simulink model "KD_cl_harness_cl_ouports_added"  (R2015b)
settings: Solver=ode45  StartTime=0  StopTime=inf  FixedStep=0.01  MaxStep=0.005  RelTol=1e-5  AbsTol=1e-5
undefined symbols (not defined in the file or in its folder): A2, bin_vec, c_0, c_1000, c_1000inv, c_100inv, c_1d2p4, c_1p7, c_4400inv, c_5500inv, c_80, c_compmap, c_ctok, c_fflow_max, c_fflow_min, c_filt, c_flowdiv, c_flowmin, c_flowmult, c_inf, c_km1d2k, c_n1, c_p00001, c_p01, c_p1e9, c_p4d1p4, c_pincomp, c_rair, c_roacorr, c_rpmtoradpers, c_svrthrottle1, c_svrthrottle2, c_svrthrottlearg, c_svrthrottlebeta, c_vnliftmax, c_vnliftmin, cl_offset, clff, Coefs, const, const_exhat, const_vec, Dual_array, dual_zero, egr_ecu_ff, expcon, f_mat, gs_jul, HQP_eps, HQP_INF, HQP_saturation, IV, L2, length_L, maxL, mHQP_saturation, minL, Newton, nRed, num_constraints ... (+22)
libraries: simulink x33
(part 2 of 6)

== system KD_cl_harness_cl_ouports_added/ambient_and_controls_in ==
  Bus Creator1 : BusCreator  Inputs=6
  From Workspace11 : FromWorkspace  VariableName="[0   97.4216]"  SampleTime=0  Interpolate=off  OutputAfterFinalValue=Holding final value
  From Workspace12 : FromWorkspace  VariableName="[0  296.9595]"  SampleTime=0  Interpolate=off  OutputAfterFinalValue=Holding final value
  From Workspace5 : FromWorkspace  VariableName="[0   97.4450]"  SampleTime=0  Interpolate=off  OutputAfterFinalValue=Holding final value
  From Workspace6 : FromWorkspace  VariableName="[0  300.0250]"  SampleTime=0  Interpolate=off  OutputAfterFinalValue=Holding final value
  From Workspace7 : FromWorkspace  VariableName="[0  351.4714]"  SampleTime=0  Interpolate=off  OutputAfterFinalValue=Holding final value
  From Workspace8 : FromWorkspace  VariableName="[0    3.7702]"  SampleTime=0  Interpolate=off  OutputAfterFinalValue=Holding final value
  ambient_in : Outport
  wires:
  Bus Creator1/1 -> ambient_in/1  "ambient_in"
  From Workspace11/1 -> Bus Creator1/1  "p_in_comp_data"
  From Workspace5/1 -> Bus Creator1/2  "p_ambient"
  From Workspace12/1 -> Bus Creator1/3  "T_in_comp_data"
  From Workspace6/1 -> Bus Creator1/4  "T_ambient"
  From Workspace7/1 -> Bus Creator1/5  "T_coolant"
  From Workspace8/1 -> Bus Creator1/6  "Tq_load"

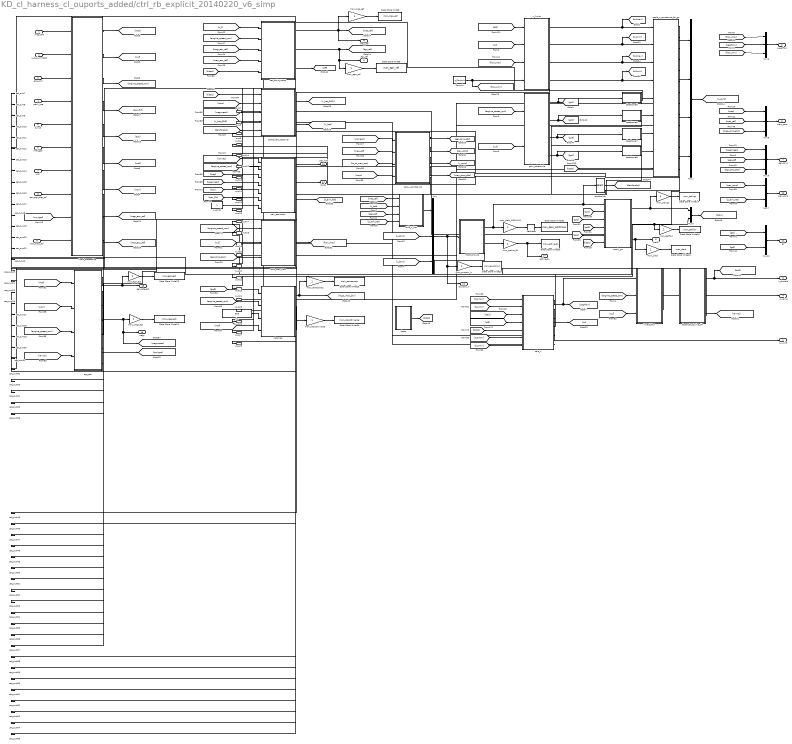
== system KD_cl_harness_cl_ouports_added/ctrl_rb_explicit_20140220_v6_simp ==
  map_kPa : Inport  OutDataTypeStr=single  PortDimensions=1  SampleTime=sample_time
  u_fuel_mm3pst : Inport  Port=2  OutDataTypeStr=single  PortDimensions=1  SampleTime=sample_time
  ene_rpm : Inport  Port=3  OutDataTypeStr=single  PortDimensions=1  SampleTime=sample_time
  pexh_kpa : Inport  Port=4  OutDataTypeStr=single  PortDimensions=1  SampleTime=sample_time
  t_in_C : Inport  Port=5  OutDataTypeStr=single  PortDimensions=1  SampleTime=sample_time
  maf_gps : Inport  Port=6  OutDataTypeStr=single  PortDimensions=1  SampleTime=sample_time
  wcyl : Inport  Port=7  OutDataTypeStr=single  PortDimensions=1  SampleTime=sample_time
  ecu_egr_rate_ref : Inport  Port=8  OutDataTypeStr=single  PortDimensions=1  SampleTime=sample_time
  ecu_map_ref : Inport  Port=9  OutDataTypeStr=single  PortDimensions=1  SampleTime=sample_time
  Data Store Write14 : DataStoreWrite  DataStoreName=mon_delvgt
  Data Store Write15 : DataStoreWrite  DataStoreName=mon_delflow
  Data Store Write16 : DataStoreWrite  DataStoreName=mon_slack
  Data Store Write23 : DataStoreWrite  DataStoreName=mon_egrr_est
  Data Store Write24 : DataStoreWrite  DataStoreName=mon_wegr_est
  Data Store Write25 : DataStoreWrite  DataStoreName=mon_remapmap
  Data Store Write29 : DataStoreWrite  DataStoreName=mon_expcon_in
  Data Store Write30 : DataStoreWrite  DataStoreName=mon_active_SL
  Data Store Write31 : DataStoreWrite  DataStoreName=mon_delU_HQPKWIK
  Data Store Write34 : DataStoreWrite  DataStoreName=mon_wtpostinverse
  Data Store Write8 : DataStoreWrite  DataStoreName=mon_map_ref
  Data Store Write9 : DataStoreWrite  DataStoreName=mon_egrr_ref
  EGR_max_flow : Subsystem
  HQPKWIK_V6 : Subsystem
  Mux{,6,8..9} (4 alike) : Mux  Inputs=3
  Mux1 : Mux
  Mux10 : Mux  Inputs=2
  Mux5 : Mux  Inputs=2
  Mux7 : Mux  Inputs=2
  Reshape : Reshape
  apply_gs : Subsystem
  calc_u : Subsystem
  calc_y_constraints : Subsystem
  constraints : Selector  InputPortWidth=3  IndexOptions=Index vector (dialog)  Indices=[1 2]  OutputSizes=1
  deadzone5 : Subsystem
  deadzone6 : Subsystem
  deadzone7 : Subsystem
  deadzone8 : Subsystem
  deconstruct_vlve_thr : Subsystem
  egr_est : Subsystem
  flowmin : Constant  Value=c_flowmin  OutDataTypeStr=single  SampleTime=sample_time
      settings: AttributesFormatString=%<Value>\n%<SampleTime>
  gain_schechule : Subsystem
  input_processing : Subsystem
  invert_flow : Subsystem  SystemSampleTime=.032
  mon_active_SL : Gain  OutDataTypeStr=int32
  mon_delU_HQPKWIK : Gain  OutDataTypeStr=single
  mon_delflow : Gain
  mon_delvgt : Gain
  mon_egrr_est : Gain
  mon_egrr_ref : Gain
  mon_expcon_in : Gain  OutDataTypeStr=single
  mon_map_ref : Gain
  mon_remapmap : Gain
  mon_slack : Gain
  mon_wegr_est : Gain
  mon_wtpostinverse : Gain
  ntremap : Subsystem  SystemSampleTime=.016
  pex_estimator : Subsystem
  scale_u_constraints_for_gs : Subsystem
  scheduled_observer : Subsystem
  set_point_maps : Subsystem
  shift_x_hat : Subsystem
  tic : Constant  Value=303  OutDataTypeStr=single  SampleTime=sample_time
      settings: AttributesFormatString=%<Value>\n%<SampleTime>
  tictoc : Subsystem
  u_limits : Subsystem
  y_cons1 : Constant  OutDataTypeStr=single  SampleTime=sample_time
      settings: AttributesFormatString=%<Value>\n%<SampleTime>
  u_vnlift : Outport  OutDataTypeStr=single
  u_egrflow : Outport  Port=2  OutDataTypeStr=single
  u_throttle : Outport  Port=3  OutDataTypeStr=single
  u_valve : Outport  Port=4  OutDataTypeStr=single
  slack : Outport  Port=5  OutDataTypeStr=single
  map_cons : Outport  Port=6  OutDataTypeStr=single
  egr_cons : Outport  Port=7  OutDataTypeStr=single
  map_ref : Outport  Port=8  OutDataTypeStr=single
  egr_ref : Outport  Port=9  OutDataTypeStr=single
  pex_cons : Outport  Port=10  OutDataTypeStr=single
  gs : Outport  Port=11  OutDataTypeStr=single
  expcon_in : Outport  Port=12  OutDataTypeStr=single
  pex_hat : Outport  Port=13  OutDataTypeStr=single
  dwdp : Outport  Port=14  OutDataTypeStr=single
  egr_rate_est : Outport  Port=15  OutDataTypeStr=single
  wegr : Outport  Port=16  OutDataTypeStr=single
  active_SL : Outport  Port=17  OutDataTypeStr=int32  PortDimensions=1
  sat_out-7 : Outport  Port=18
  sat_out-8 : Outport  Port=19
  sat_out-9 : Outport  Port=20
  sat_out-10 : Outport  Port=21
  sat_out-11 : Outport  Port=22
  sat_out-12 : Outport  Port=23
  sat_out-13 : Outport  Port=24
  sat_out-14 : Outport  Port=25
  sat_out-15 : Outport  Port=26
  sat_out-16 : Outport  Port=27
  sat_out-17 : Outport  Port=28
  sat_out-18 : Outport  Port=29
  sat_out-19 : Outport  Port=30
  sat_out-20 : Outport  Port=31
  sat_out-21 : Outport  Port=32
  sat_out-22 : Outport  Port=33
  sat_out-23 : Outport  Port=34
  sat_out-24 : Outport  Port=35
  sat_out-25 : Outport  Port=36
  sat_out-26 : Outport  Port=37
  sat_out-27 : Outport  Port=38
  sat_out-28 : Outport  Port=39
  sat_out-29 : Outport  Port=40
  sat_out-30 : Outport  Port=41
  sat_out-31 : Outport  Port=42
  sat_out-32 : Outport  Port=43
  sat_out-33 : Outport  Port=44
  sat_out-34 : Outport  Port=45
  sat_out-35 : Outport  Port=46
  sat_out-36 : Outport  Port=47
  sat_out-45 : Outport  Port=48
  sat_out-46 : Outport  Port=49
  sat_out-47 : Outport  Port=50
  sat_out-48 : Outport  Port=51
  sat_out-49 : Outport  Port=52
  sat_out-50 : Outport  Port=53
  sat_out-51 : Outport  Port=54
  sat_out-52 : Outport  Port=55
  sat_out-53 : Outport  Port=56
  sat_out-54 : Outport  Port=57
  sat_out-55 : Outport  Port=58
  sat_out-56 : Outport  Port=59
  sat_out-57 : Outport  Port=60
  sat_out-58 : Outport  Port=61
  sat_out-59 : Outport  Port=62
  sat_out-60 : Outport  Port=63
  sat_out-61 : Outport  Port=64
  sat_out-62 : Outport  Port=65
  sat_out-63 : Outport  Port=66
  sat_out-64 : Outport  Port=67
  sat_out-65 : Outport  Port=68
  out-7 : Outport  Port=69
  out-8 : Outport  Port=70
  out-9 : Outport  Port=71
  out-10 : Outport  Port=72
  out-11 : Outport  Port=73
  out-12 : Outport  Port=74
  out-13 : Outport  Port=75
  out-14 : Outport  Port=76
  out-15 : Outport  Port=77
  out-16 : Outport  Port=78
  out-17 : Outport  Port=79
  out-18 : Outport  Port=80
  out-19 : Outport  Port=81
  out-20 : Outport  Port=82
  out-21 : Outport  Port=83
  out-22 : Outport  Port=84
  out-23 : Outport  Port=85
  out-24 : Outport  Port=86
  out-25 : Outport  Port=87
  out-26 : Outport  Port=88
  out-27 : Outport  Port=89
  out-28 : Outport  Port=90
  wires:
  [tu2min] -> calc_u/7(tu2min)
  [tu2max] -> calc_u/6(tu2max)
  [tu1min] -> calc_u/2(tu1min)
  [tu1max] -> calc_u/1(tu1max)
  [wt_to_map_con] -> calc_y_constraints/3(wt_to_map_con)
  [map] -> calc_y_constraints/4(map)
  ntremap/2(wtinv) -> mon_wtpostinverse/1
  mon_wtpostinverse/1 -> Data Store Write34/1
  [map_ecu_ref] -> set_point_maps/4(map_ecu_ref)
  [wegr_ecu_ref] -> set_point_maps/3(wegr_ecu_ref)
  [wcylgps] -> input_processing/9(wcylgps)
  egr_est/3(wcylgps) -> [wcylgps]
  ecu_map_ref/1 -> input_processing/10(ecu_map_ref)
  [w_f] -> gain_schechule/2(qv)
  [engine_speed_rpm] -> gain_schechule/1(ene)
  mon_remapmap/1 -> Data Store Write25/1
  ntremap/1(mapconsremaped) -> mon_remapmap/1, [wt_to_map_con]
  [tictoc] -> calc_u/5(tictoc)
  deadzone8/1(Out1) -> scale_u_constraints_for_gs/8(gs4)
  deadzone7/1(Out1) -> scale_u_constraints_for_gs/7(gs3)
  deadzone6/1(Out1) -> scale_u_constraints_for_gs/6(gs2)
  deadzone5/1(Out1) -> scale_u_constraints_for_gs/5(gs1)
  constraints/1 -> [deluforobs]
  [tictoc] -> scheduled_observer/1(tictoc)
  gain_schechule/4(gs4) -> [gs4], deadzone8/1(In1)
  gain_schechule/2(gs2) -> [gs2], deadzone6/1(In1)
  gain_schechule/1(gs1) -> [gs1], deadzone5/1(In1)
  scheduled_observer/1(xhatRO) -> [x_hat_ROO]
  scheduled_observer/2(xhat) -> [x_hat]
  Reshape/1 -> Data Store Write31/1
  mon_delU_HQPKWIK/1 -> Reshape/1
  calc_u/3(u_unlift) -> u_vnlift/1
  Mux/1 -> expcon_in/1, mon_expcon_in/1, HQPKWIK_V6/1(u)
  [y_cons] -> Mux/3
  Mux5/1 -> [delu]
  [u_cons] -> Mux/2
  [engine_speed_rpm] -> EGR_max_flow/1(Ne_rpm)
  [map_ref] -> shift_x_hat/1(map_ref)
  [egr_ref] -> shift_x_hat/3(egr_ref)
  [x_hat] -> shift_x_hat/2(x_hat)
  [wegrmeas] -> Mux9/1
  [map_ref] -> Mux8/2
  [map] -> Mux8/1
  Mux9/1 -> egr_cons/1
  Mux8/1 -> map_cons/1
  [flow_min] -> Mux6/3
  [flow_max] -> Mux6/1
  Mux6/1 -> u_egrflow/1
  [egr_ref] -> Mux9/2
  [engine_speed_rpm] -> invert_flow/2(ne_rpm)
  ene_rpm/1 -> input_processing/3(Ne)
  flowmin/1 -> [flow_min], u_limits/4(flow_min)
  u_fuel_mm3pst/1 -> input_processing/2(fuel)
  set_point_maps/1(intake_pressure_ref) -> [map_ref], map_ref/1, mon_map_ref/1
  set_point_maps/2(EGR_ref) -> [egr_ref], egr_ref/1, mon_egrr_ref/1
  [w_f] -> set_point_maps/1(fuel_rate_mm3perst)
  [engine_speed_rpm] -> set_point_maps/2(engine_speed_rpm)
  [delu] -> calc_u/3(delu)
  [map_cons_abs] -> Mux8/3
  [egr_cons_abs] -> Mux9/3
  [p_exh_hat] -> shift_x_hat/4(pex_hat)
  Mux7/1 -> pex_cons/1
  [pex_cons] -> Mux7/1
  [p_exh_hat] -> Mux7/2
  [gs1] -> Mux10/1
  [gs2] -> Mux10/2
  Mux10/1 -> gs/1
  input_processing/5(tico) -> [tico]
  maf_gps/1 -> input_processing/6(maf_gps)
  deconstruct_vlve_thr/3(valvez) -> [valvez]
  wcyl/1 -> input_processing/7(wcyl_gps)
  [maf] -> egr_est/1(maf)
  [wcyl] -> egr_est/2(wcyl)
  [engine_speed_rpm] -> egr_est/3(ene)
  egr_est/1(egrr) -> egr_rate_est/1, mon_egrr_est/1
  egr_est/2(wegr) -> [wegrmeas], wegr/1, mon_wegr_est/1
  [wegrmeas] -> scheduled_observer/3(egrr)
  [map] -> scheduled_observer/2(map)
  [deluforobs] -> scheduled_observer/5(u)
  [x_hat_ROO] -> scheduled_observer/4(xhatROpm1)
  [valvez] -> egr_est/4(valve)
  [valvez] -> pex_estimator/1(valvez)
  [engine_speed_rpm] -> pex_estimator/2(Ne_rpm)
  [map] -> pex_estimator/3(map)
  [wegrmeas] -> pex_estimator/4(wegr)
  [tico] -> pex_estimator/5(tico)
  [pex_filt] -> pex_estimator/6(pex_filt)
  pex_estimator/1(pex_hat) -> pex_hat/1
  pex_estimator/2(dwdp) -> dwdp/1
  y_cons1/1 -> pex_estimator/7(while)
  tic/1 -> ntremap/3(T_out_IC)
  [engine_speed_rpm] -> ntremap/2(omega_engine_rpm)
  [thrff] -> ntremap/1(u_EGR_throttle)
  [maf] -> ntremap/4(maf)
  mon_egrr_est/1 -> Data Store Write23/1
  mon_wegr_est/1 -> Data Store Write24/1
  mon_map_ref/1 -> Data Store Write8/1
  mon_egrr_ref/1 -> Data Store Write9/1
  mon_slack/1 -> Data Store Write16/1
  mon_delflow/1 -> Data Store Write15/1
  mon_delvgt/1 -> Data Store Write14/1
  [uegrflow] -> Mux6/2
  scale_u_constraints_for_gs/4(gsu2min) -> Mux1/4
  scale_u_constraints_for_gs/3(gsu2max) -> Mux1/3
  scale_u_constraints_for_gs/2(gsu1min) -> Mux1/2
  scale_u_constraints_for_gs/1(gsu1max) -> Mux1/1
  [tictoc] -> scale_u_constraints_for_gs/9(tictoc)
  calc_y_constraints/3(y_cons) -> [y_cons]
  Mux1/1 -> [u_cons]
  [flow_max] -> u_limits/3(flow_max)
  [gs1] -> apply_gs/2(gs1)
  [gs2] -> apply_gs/3(gs2)
  [gs3] -> apply_gs/4(gs3)
  [gs4] -> apply_gs/5(gs4)
  [tictoc] -> apply_gs/6(tictoc)
  apply_gs/1(delu1) -> Mux5/1, mon_delvgt/1
  apply_gs/2(delu2) -> Mux5/2, mon_delflow/1
  apply_gs/3(slack) -> mon_slack/1, slack/1
  u_limits/1(u1max) -> [tu1max], scale_u_constraints_for_gs/1(u1max)
  u_limits/2(u1min) -> [tu1min], scale_u_constraints_for_gs/2(u1min)
  u_limits/3(u2max) -> [tu2max], scale_u_constraints_for_gs/3(u2max)
  u_limits/4(u2min) -> [tu2min], scale_u_constraints_for_gs/4(u2min)
  mon_active_SL/1 -> Data Store Write30/1, active_SL/1
  input_processing/4(pex_filt) -> [pex_filt]
  mon_expcon_in/1 -> Data Store Write29/1
  deconstruct_vlve_thr/1(u_throttle) -> u_throttle/1, [thrff]
  [w_f] -> EGR_max_flow/2(fuel)
  [w_f] -> invert_flow/3(qv_mm3st)
  [uz] -> u_limits/2(uz)
  [clff] -> u_limits/1(clff)
  [clff] -> calc_u/4(clff)
  HQPKWIK_V6/1(delU) -> mon_delU_HQPKWIK/1, apply_gs/1(ustar), constraints/1
  HQPKWIK_V6/2(SL_sum) -> mon_active_SL/1
  EGR_max_flow/1(egr_flow_max) -> [flow_max]
  tictoc/1(tictoc) -> [tictoc]
  [wcylgps] -> calc_y_constraints/1(wcylgps)
  calc_y_constraints/1(egr_cons_abs) -> [egr_cons_abs]
  [egr_cons_abs] -> EGR_max_flow/3(egr_cons_abs)
  [tictoc] -> set_point_maps/5(tictoc)
  set_point_maps/3(clff) -> [clff]
  pex_estimator/3(pex_hat_limited) -> [p_exh_hat]
  shift_x_hat/1(x_hat_shift) -> Mux/1
  calc_y_constraints/2(pex_cons) -> [pex_cons]
  calc_y_constraints/4(map_cons_abs) -> [map_cons_abs]
  [map_ref] -> calc_y_constraints/2(map_ref)
  calc_u/2(uz) -> [uz]
  calc_u/1(uegrflow) -> [uegrflow], invert_flow/1(valve_flow_command)
  invert_flow/1(uvalve) -> deconstruct_vlve_thr/1(uvalve)
  deconstruct_vlve_thr/2(u_valve) -> u_valve/1
  pexh_kpa/1 -> input_processing/4(In3)
  t_in_C/1 -> input_processing/5(t_in_C)
  ecu_egr_rate_ref/1 -> input_processing/8(ecu_egr_rate_ref)
  input_processing/8(wegr_ecu_ref) -> [wegr_ecu_ref]
  input_processing/9(map_ecu_ref) -> [map_ecu_ref]
  input_processing/7(wcyl) -> [wcyl]
  input_processing/6(maf) -> [maf]
  input_processing/3(Ne_rpm) -> [engine_speed_rpm]
  input_processing/2(w_f) -> [w_f]
  input_processing/1(map) -> [map]
  map_kPa/1 -> input_processing/1(map_kpa)
  gain_schechule/3(gs3) -> deadzone7/1(In1), [gs3]
  EGR_max_flow/2(sat_out-7) -> sat_out-7/1
  HQPKWIK_V6/3(sat_out-8) -> sat_out-8/1
  HQPKWIK_V6/4(sat_out-9) -> sat_out-9/1
  calc_u/4(sat_out-10) -> sat_out-10/1
  calc_y_constraints/5(sat_out-11) -> sat_out-11/1
  deadzone5/2(sat_out-12) -> sat_out-12/1
  deadzone6/2(sat_out-13) -> sat_out-13/1
  deadzone7/2(sat_out-14) -> sat_out-14/1
  deadzone8/2(sat_out-15) -> sat_out-15/1
  deconstruct_vlve_thr/4(sat_out-16) -> sat_out-16/1
  egr_est/4(sat_out-17) -> sat_out-17/1
  egr_est/5(sat_out-18) -> sat_out-18/1
  input_processing/10(sat_out-19) -> sat_out-19/1
  invert_flow/2(sat_out-20) -> sat_out-20/1
  ntremap/3(sat_out-21) -> sat_out-21/1
  set_point_maps/4(sat_out-22) -> sat_out-22/1
  set_point_maps/5(sat_out-23) -> sat_out-23/1
  u_limits/5(sat_out-24) -> sat_out-24/1
  egr_est/6(sat_out-25) -> sat_out-25/1
  egr_est/7(sat_out-26) -> sat_out-26/1
  ntremap/4(sat_out-27) -> sat_out-27/1
  ntremap/5(sat_out-28) -> sat_out-28/1
  ntremap/6(sat_out-29) -> sat_out-29/1
  ntremap/7(sat_out-30) -> sat_out-30/1
  pex_estimator/4(sat_out-31) -> sat_out-31/1
  pex_estimator/5(sat_out-32) -> sat_out-32/1
  pex_estimator/6(sat_out-33) -> sat_out-33/1
  pex_estimator/7(sat_out-34) -> sat_out-34/1
  pex_estimator/8(sat_out-35) -> sat_out-35/1
  pex_estimator/9(sat_out-36) -> sat_out-36/1
  ntremap/8(sat_out-45) -> sat_out-45/1
  ntremap/9(sat_out-46) -> sat_out-46/1
  pex_estimator/10(sat_out-47) -> sat_out-47/1
  pex_estimator/11(sat_out-48) -> sat_out-48/1
  pex_estimator/12(sat_out-49) -> sat_out-49/1
  pex_estimator/13(sat_out-50) -> sat_out-50/1
  pex_estimator/14(sat_out-51) -> sat_out-51/1
  pex_estimator/15(sat_out-52) -> sat_out-52/1
  pex_estimator/16(sat_out-53) -> sat_out-53/1
  pex_estimator/17(sat_out-54) -> sat_out-54/1
  pex_estimator/18(sat_out-55) -> sat_out-55/1
  pex_estimator/19(sat_out-56) -> sat_out-56/1
  pex_estimator/20(sat_out-57) -> sat_out-57/1
  ntremap/10(sat_out-58) -> sat_out-58/1
  ntremap/11(sat_out-59) -> sat_out-59/1
  ntremap/12(sat_out-60) -> sat_out-60/1
  ntremap/13(sat_out-61) -> sat_out-61/1
  ntremap/14(sat_out-62) -> sat_out-62/1
  ntremap/15(sat_out-63) -> sat_out-63/1
  ntremap/16(sat_out-64) -> sat_out-64/1
  ntremap/17(sat_out-65) -> sat_out-65/1
  apply_gs/4(out-7) -> out-7/1
  calc_u/5(out-8) -> out-8/1
  scale_u_constraints_for_gs/5(out-9) -> out-9/1
  scale_u_constraints_for_gs/6(out-10) -> out-10/1
  scale_u_constraints_for_gs/7(out-11) -> out-11/1
  scale_u_constraints_for_gs/8(out-12) -> out-12/1
  scale_u_constraints_for_gs/9(out-13) -> out-13/1
  set_point_maps/6(out-14) -> out-14/1
  set_point_maps/7(out-15) -> out-15/1
  set_point_maps/8(out-16) -> out-16/1
  ntremap/18(out-17) -> out-17/1
  apply_gs/5(out-18) -> out-18/1
  calc_u/6(out-19) -> out-19/1
  scale_u_constraints_for_gs/10(out-20) -> out-20/1
  scale_u_constraints_for_gs/11(out-21) -> out-21/1
  scale_u_constraints_for_gs/12(out-22) -> out-22/1
  scale_u_constraints_for_gs/13(out-23) -> out-23/1
  scale_u_constraints_for_gs/14(out-24) -> out-24/1
  set_point_maps/9(out-25) -> out-25/1
  set_point_maps/10(out-26) -> out-26/1
  set_point_maps/11(out-27) -> out-27/1
  ntremap/19(out-28) -> out-28/1

== system KD_cl_harness_cl_ouports_added/pre-throttle manifold ==
  compressor_out : Inport
  intercooler_out : Inport  Port=2
  egr_throttle_out : Inport  Port=3
  Intake_man_out : Inport  Port=4
  Bus Creator : BusCreator  Inputs=1
  Bus Creator1 : BusCreator  Inputs=4
  Bus Selector : BusSelector  OutputSignals=compressor_out.W_compressor,egr_throttle_out.W_EGR_Throttle,compressor_out.T_out_comp_sim,intercooler_out.T_out_IC
  p_preThrottle : Subsystem
  pre_throttle_out : Outport
  p_pre_throttle : Outport  Port=2
  wires:
  Bus Creator/1 -> pre_throttle_out/1  "pre_throttle_out"
  p_preThrottle/1("p_pre_throttle ") -> Bus Creator/1, p_pre_throttle/1  "p_pre_throttle"
  compressor_out/1 -> Bus Creator1/1
  intercooler_out/1 -> Bus Creator1/2
  egr_throttle_out/1 -> Bus Creator1/3
  Bus Creator1/1 -> Bus Selector/1
  Bus Selector/1 -> p_preThrottle/1(W_compressor)  "<W_compressor>"
  Bus Selector/2 -> p_preThrottle/2(W_throttle)  "<W_EGR_Throttle>"
  Bus Selector/3 -> p_preThrottle/3(T_out_compressor)  "<T_out_comp_sim>"
  Bus Selector/4 -> p_preThrottle/4(T_out_IC_data)  "<T_out_IC>"
  Intake_man_out/1 -> Bus Creator1/4

== system KD_cl_harness_cl_ouports_added/steps ==
  Constant : Constant
  Constant1 : Constant
  Constant2 : Constant  Value=2500
  From Workspace : FromWorkspace  VariableName=[0 5;10 55;20 5]  SampleTime=0  Interpolate=off  OutputAfterFinalValue=Holding final value
  Manual Switch : ManualSwitch  CurrentSetting=0
  Manual Switch1 : ManualSwitch
  Mux1 : Mux  Inputs=2
  Mux2 : Mux  Inputs=2
  Mux3 : Mux  Inputs=2
  Ne : simulink/Math Operations/Slider Gain  low=800  gain=2500  high=4000
  Subsystem : Subsystem  TreatAsAtomicUnit=on  SystemSampleTime=.032
  Subsystem1 : Subsystem  TreatAsAtomicUnit=on  SystemSampleTime=.032
  Subsystem2 : Subsystem  TreatAsAtomicUnit=on  SystemSampleTime=.032
  Uniform Random Number : UniformRandomNumber  Minimum=0  Maximum=60  SampleTime=5
  Uniform Random Number1 : UniformRandomNumber  Minimum=1000  Maximum=4000  SampleTime=50
  W_f : simulink/Math Operations/Slider Gain  low=0  gain=60  high=60
  Out1 : Outport
  wires:
  Constant/1 -> Ne/1
  Constant1/1 -> W_f/1
  W_f/1 -> Mux2/1
  Ne/1 -> Mux2/2
  Uniform Random Number1/1 -> Subsystem1/1(In1)
  Mux2/1 -> Manual Switch/1
  Mux1/1 -> Manual Switch/2
  Uniform Random Number/1 -> Subsystem/1(In1)
  Subsystem/1(Out1) -> Mux1/1
  Subsystem1/1(Out1) -> Mux1/2
  Manual Switch/1 -> Manual Switch1/1
  Manual Switch1/1 -> Out1/1
  Constant2/1 -> Mux3/2
  Subsystem2/1(Out1) -> Mux3/1
  From Workspace/1 -> Subsystem2/1(In1)
  Mux3/1 -> Manual Switch1/2

== system KD_cl_harness_cl_ouports_added/Combsution/Exhaust  ==
  omega_engine_radS : Inport
  T_intake_man : Inport  Port=2
  W_cyl : Inport  Port=3
  u_fuel : Inport  Port=4
  F1_in_man : Inport  Port=5
  Constant3 : Constant  Value=Coefs.ExhaustTemp
  MATLAB Function1 : MATLAB Function  TreatAsAtomicUnit=on
  conversion to RPM : Gain  Gain=30/pi
  T_exhaust : Outport
  wires:
  MATLAB Function1/1(T_exhaust) -> T_exhaust/1
  omega_engine_radS/1 -> conversion to RPM/1
  u_fuel/1 -> MATLAB Function1/4(u_fuel)
  F1_in_man/1 -> MATLAB Function1/5(F1_in)
  Constant3/1 -> MATLAB Function1/6(ExhaustTempCoefs)
  conversion to RPM/1 -> MATLAB Function1/1(omega_engine_rpm)
  T_intake_man/1 -> MATLAB Function1/2(T_in_man)
  W_cyl/1 -> MATLAB Function1/3(W_cyl)

== system KD_cl_harness_cl_ouports_added/Combsution/cylinder comp ==
  omega_engine_radS : Inport
  p_intake_man : Inport  Port=2
  p_exhaust_man : Inport  Port=3
  T_intake_man : Inport  Port=4
  T_exhaust_man : Inport  Port=5
  Constant : Constant  Value=const.Engine_Displacement_Volume_m3
  Constant1 : Constant  Value=const.R_specific_air_KJ_per_kg_kelvin
  Constant2 : Constant  Value=Coefs.CylFlow
  MATLAB Function : MATLAB Function  Priority=1  TreatAsAtomicUnit=on
  Mux : Mux  Inputs=2
  Terminator_3 : Terminator
  conversion to RPM : Gain  Gain=30/pi
  W_cyl_sim : Outport
  wires:
  Constant/1 -> Mux/1
  Mux/1 -> MATLAB Function/6(CylConstants)
  Constant1/1 -> Mux/2
  MATLAB Function/1(W_cyl_out) -> W_cyl_sim/1
  Constant2/1 -> MATLAB Function/7(cylFlowCoefs)
  omega_engine_radS/1 -> conversion to RPM/1
  conversion to RPM/1 -> MATLAB Function/1(omega_engine)
  p_intake_man/1 -> MATLAB Function/2(p_in_man)
  p_exhaust_man/1 -> MATLAB Function/3(p_exh_man)
  T_intake_man/1 -> MATLAB Function/4(T_in_man)
  T_exhaust_man/1 -> MATLAB Function/5(T_exh_man)
  MATLAB Function/2(nVol) -> Terminator_3/1

== system KD_cl_harness_cl_ouports_added/Compressor/Comp Map ==
  p_in_comp : Inport
  p_out_comp : Inport  Port=2
  T_in_comp_data : Inport  Port=3
  omega_turbo_data_radS : Inport  Port=4
  Constant : Constant  Value=const.compressor_diameter
  Constant1 : Constant  Value=const.Cp_Air_300K_J_per_kg_per_K
  Constant2 : Constant  Value=const.rho_Air_300K_kg_per_m3
  Constant3 : Constant  Value=const.gamma_air
  Constant4 : Constant  Value=const.R_specific_air_J_per_kg_kelvin
  Constant5 : Constant  Value=Coefs.CompPresRat
  Constant6 : Constant  Value=Coefs.CompEff
  Divide : Product  Inputs=/*
  MATLAB Function : MATLAB Function  TreatAsAtomicUnit=on
  Mux : Mux  Inputs=5
  Mux1 : Mux  Inputs=13
      settings: DisplayOption=signals
  Terminator_1 : Terminator
  Terminator_3 : Terminator
  conversion to RPM : Gain  Gain=30/pi
  W_comp_sim : Outport
  T_out_comp_sim : Outport  Port=2
  Tq_comp : Outport  Port=3
  wires:
  Mux/1 -> MATLAB Function/4(Comp_Constants)
  Constant5/1 -> MATLAB Function/5(CompPresRatCoefs)
  Constant6/1 -> MATLAB Function/6(CompEffCoefs)
  MATLAB Function/1(W_comp) -> W_comp_sim/1
  MATLAB Function/2(T_out_comp) -> T_out_comp_sim/1
  MATLAB Function/17(Tq_Compressor) -> Tq_comp/1
  MATLAB Function/4(pres_Rat1) -> Mux1/1
  MATLAB Function/5(Uc) -> Mux1/2
  MATLAB Function/6(Mach) -> Mux1/3
  MATLAB Function/7(psi) -> Mux1/4
  MATLAB Function/8(k1) -> Mux1/5
  MATLAB Function/9(k2) -> Mux1/6
  MATLAB Function/10(k3) -> Mux1/7
  MATLAB Function/11(PhiC) -> Mux1/8
  MATLAB Function/12(Comp_Efficiency) -> Mux1/9
  MATLAB Function/13(PhiC1) -> Mux1/10
  MATLAB Function/14(a1) -> Mux1/11
  MATLAB Function/15(a2) -> Mux1/12
  MATLAB Function/16(a3) -> Mux1/13
  p_in_comp/1 -> Divide/1
  p_out_comp/1 -> Divide/2
  Divide/1 -> MATLAB Function/1(pres_Rat)
  T_in_comp_data/1 -> MATLAB Function/2(T_in_comp)
  omega_turbo_data_radS/1 -> conversion to RPM/1
  conversion to RPM/1 -> MATLAB Function/3(omega_turbo_RPM)
  Constant/1 -> Mux/1
  Constant3/1 -> Mux/2
  Constant4/1 -> Mux/3
  Constant1/1 -> Mux/4
  Constant2/1 -> Mux/5
  Mux1/1 -> Terminator_1/1
  MATLAB Function/3(P_comp_W) -> Terminator_3/1

== system KD_cl_harness_cl_ouports_added/EGR Throttle/EGR Throttle ==
  u_EGR_throttle : Inport
  omega_engine_radS : Inport  Port=2
  p_intake_man : Inport  Port=3
  T_out_IC : Inport  Port=4
  p_preThrottle : Inport  Port=5
  Gain : Gain  Gain=1000
  Gain1 : Gain  Gain=1000
  Saturation : Saturate  UpperLimit=1  LowerLimit=0.001
  Terminator : Terminator
  Terminator1 : Terminator
  Throttle Model2 : Subsystem
  conversion to RPM : Gain  Gain=30/pi
  ThrottleFlow_kgpers : Outport
  sat_out-6 : Outport  Port=2
  sat_out-37 : Outport  Port=3
  sat_out-38 : Outport  Port=4
  sat_out-39 : Outport  Port=5
  sat_out-40 : Outport  Port=6
  out-1 : Outport  Port=7
  out-3 : Outport  Port=8
  out-4 : Outport  Port=9
  wires:
  Throttle Model2/1(mt[kg/sec]) -> Saturation/1, sat_out-6/1
  Throttle Model2/2(forwardmt[kg/sec]) -> Terminator/1
  u_EGR_throttle/1 -> Throttle Model2/1(TA[deg])
  omega_engine_radS/1 -> conversion to RPM/1
  p_intake_man/1 -> Gain/1
  T_out_IC/1 -> Throttle Model2/4(Tim[K]), Throttle Model2/6(Tamb[K])
  p_preThrottle/1 -> Gain1/1
  conversion to RPM/1 -> Throttle Model2/2(Ne[rpm])
  Gain/1 -> Throttle Model2/3(Pim[Pa])
  Gain1/1 -> Throttle Model2/5(Pamb[Pa])
  Throttle Model2/3(backwardmt[kg/sec]) -> Terminator1/1
  Saturation/1 -> ThrottleFlow_kgpers/1
  Throttle Model2/4(sat_out-37) -> sat_out-37/1
  Throttle Model2/5(sat_out-38) -> sat_out-38/1
  Throttle Model2/6(sat_out-39) -> sat_out-39/1
  Throttle Model2/7(sat_out-40) -> sat_out-40/1
  Throttle Model2/8(out-1) -> out-1/1
  Throttle Model2/9(out-3) -> out-3/1
  Throttle Model2/10(out-4) -> out-4/1

== system KD_cl_harness_cl_ouports_added/EGR Valve/SVR EGR ==
  u_EGR_valve : Inport
  omega_engine_data_radS : Inport  Port=2
  p_intake_man_data : Inport  Port=3
  T_out_egr_cooler : Inport  Port=4
  p_exhaust_man_data : Inport  Port=5
  EGR_model : Subsystem
  Gain1 : Gain  Gain=1000
  Gain2 : Gain  Gain=1000
  Memory : Memory  X0=IV.T_out_egr_cooler  InheritSampleTime=on
  Terminator : Terminator
  conversion to RPM : Gain  Gain=30/pi
  EGR_kgpers : Outport
  sat_out-41 : Outport  Port=2
  sat_out-42 : Outport  Port=3
  sat_out-43 : Outport  Port=4
  sat_out-44 : Outport  Port=5
  out-2 : Outport  Port=6
  out-5 : Outport  Port=7
  out-6 : Outport  Port=8
  wires:
  EGR_model/1(mt[kg/sec]) -> EGR_kgpers/1
  EGR_model/2(forwardmt[kg/sec]) -> Terminator/1
  u_EGR_valve/1 -> EGR_model/1(TA[deg])
  omega_engine_data_radS/1 -> conversion to RPM/1
  p_intake_man_data/1 -> Gain1/1
  T_out_egr_cooler/1 -> Memory/1
  p_exhaust_man_data/1 -> Gain2/1
  Gain1/1 -> EGR_model/3(Pim[Pa])
  Gain2/1 -> EGR_model/5(Pamb[Pa])
  conversion to RPM/1 -> EGR_model/2(Ne[rpm])
  Memory/1 -> EGR_model/4(Tim[K]), EGR_model/6(Tamb[K])
  EGR_model/3(sat_out-41) -> sat_out-41/1
  EGR_model/4(sat_out-42) -> sat_out-42/1
  EGR_model/5(sat_out-43) -> sat_out-43/1
  EGR_model/6(sat_out-44) -> sat_out-44/1
  EGR_model/7(out-2) -> out-2/1
  EGR_model/8(out-5) -> out-5/1
  EGR_model/9(out-6) -> out-6/1

== system KD_cl_harness_cl_ouports_added/EGR cooler/EGR Cooler ==
  note: to reduce the numerical sensitivity
  T_exh_man : Inport
  T_coolant : Inport  Port=2
  W_egr_valve : Inport  Port=3
  u_EGR_cooler_bypass : Inport  Port=4
  omega_engine_data_radS : Inport  Port=5
  T_ambient : Inport  Port=6
  Constant : Constant  Value=Coefs.EGRCoolerTemp
  Constant1 : Constant  Value=Coefs.EGRCoolerbypassTemp
  Fcn3 : Fcn  Expr="Coefs.TinEGR(1)  + Coefs.TinEGR(2)*u(1) + Coefs.TinEGR(3)*u(2) + Coefs.TinEGR(4)*u(3) + Coefs.TinEGR(5)*u(1)^2 +Coefs.TinEGR(6)*u(2)^2"
  MATLAB Function : MATLAB Function  TreatAsAtomicUnit=on
  Mux3 : Mux  Inputs=3
  conversion to RPM1 : Gain  Gain=30/pi
  gain : Gain  Gain=1000
  T_out_EGR_cooler_sim : Outport
  W_egr_cooler : Outport  Port=2
  wires:
  Constant/1 -> MATLAB Function/6(EGRCoolerTempCoefs)
  Constant1/1 -> MATLAB Function/7(EGRCoolerbypassTempCoefs)
  MATLAB Function/1(T_out_EGR_cooler) -> T_out_EGR_cooler_sim/1
  T_coolant/1 -> MATLAB Function/2(T_coolant)
  u_EGR_cooler_bypass/1 -> MATLAB Function/4(EGRbypassflag)
  omega_engine_data_radS/1 -> conversion to RPM1/1
  conversion to RPM1/1 -> MATLAB Function/5(engine_speed_RPM)
  Fcn3/1 -> MATLAB Function/1(T_in_EGR_cooler)
  Mux3/1 -> Fcn3/1
  T_ambient/1 -> Mux3/3
  gain/1 -> Mux3/2
  W_egr_valve/1 -> W_egr_cooler/1, MATLAB Function/3(W_egr_valve), gain/1
  T_exh_man/1 -> Mux3/1

== system KD_cl_harness_cl_ouports_added/Exhaust Manifold/Exhaust Manifold ==
  note: Total mass flow rate into the engine
  note: Total mass flow rate out of the engine
  W_egr_valve : Inport
  W_cylinder : Inport  Port=2
  u_fuel : Inport  Port=3
  W_turbine : Inport  Port=4
  F_engine_out : Inport  Port=5
  exhaust_temp : Inport  Port=6
  T_intake_man : Inport  Port=7
  T_ambient : Inport  Port=8
  " R_air" : Gain  Gain=const.R_specific_air_KJ_per_kg_kelvin
  1/exhaust manifold volume : Gain  Gain=1/Coefs.V_exhaust_man_m3
  Add1 : Sum
  Add3 : Sum  Inputs=+--
  Cus_integrator : Subsystem
  Cus_integrator1 : Subsystem
  Cus_integrator2 : Subsystem
  Divide : Product  Inputs=/*
  Divide1 : Product  Inputs=/*
  Divide2 : Product  Inputs=*/
  Fcn : Fcn  Expr=u(1)*(u(2) -u(3))
  Fcn1 : Fcn  Expr=(u(1)*u(2) -u(3)*u(6) -u(4)*u(6)) - u(7)/const.Cp_Air_300K_KJ_per_kg_per_K
  Mux : Mux  Inputs=3
  Mux1 : Mux  Inputs=7
  Product : Product  RndMeth=Zero
  Sum : Sum  Inputs=-+
  exhaust manifold volume : Gain  Gain=Coefs.V_exhaust_man_m3
  exhaust_manifold_vol : Constant  Value=Coefs.V_exhaust_man_m3
  gamma* R_air : Gain  Gain=const.gamma_air*const.R_specific_air_KJ_per_kg_kelvin
  k_heat_W : Gain  Gain=Coefs.K_heat_W
  p_exh_man_sim : Outport
  T_exh_man_sim : Outport  Port=2
  F_exh_man_sim : Outport  Port=3
  wires:
  Add1/1 -> [W_tot_out_engine]
  [W_tot_out_engine] -> Add3/1
  [W_turbine] -> Add3/2
  [W_egr_valve] -> Add3/3
  Add3/1 -> 1/exhaust manifold volume/1
  1/exhaust manifold volume/1 -> Cus_integrator/1(in)
  [W_tot_out_engine] -> Mux/1
  F_engine_out/1 -> Mux/2
  Mux/1 -> Fcn/1
  Fcn/1 -> Divide/2
  exhaust manifold volume/1 -> Divide/1
  Divide/1 -> Cus_integrator1/1(in)
  Cus_integrator1/1(F2_exhaust) -> Mux/3, F_exh_man_sim/1
  Mux1/1 -> Fcn1/1
  gamma* R_air/1 -> Divide2/1
  Fcn1/1 -> gamma* R_air/1
  Cus_integrator2/1(p_exhaust) -> p_exh_man_sim/1, Divide1/2
  " R_air"/1 -> Divide1/1
  Divide1/1 -> Mux1/6, T_exh_man_sim/1
  Divide2/1 -> Cus_integrator2/1(in)
  exhaust_manifold_vol/1 -> Divide2/2
  Cus_integrator/1(rho_exhaust) -> exhaust manifold volume/1, " R_air"/1
  [W_tot_out_engine] -> Mux1/1
  [W_turbine] -> Mux1/3
  [W_egr_valve] -> Mux1/4
  exhaust_temp/1 -> Mux1/2, Sum/2
  W_cylinder/1 -> Add1/1
  W_egr_valve/1 -> [W_egr_valve]
  u_fuel/1 -> Add1/2
  W_turbine/1 -> [W_turbine]
  T_intake_man/1 -> Mux1/5
  Product/1 -> k_heat_W/1
  T_ambient/1 -> Sum/1
  [W_tot_out_engine] -> Product/1
  Sum/1 -> Product/2
  k_heat_W/1 -> Mux1/7

== system KD_cl_harness_cl_ouports_added/Intake Manifold/Intake_manifold ==
  note: Total mass flow rate into the engine
  W_throttle : Inport
  W_egr_valve : Inport  Port=2
  W_cyl_in : Inport  Port=3
  F2_exhaust_sim : Inport  Port=4
  T_out_egr_cooler : Inport  Port=5
  T_out_IC : Inport  Port=6
  " R_air1" : Gain  Gain=const.R_specific_air_KJ_per_kg_kelvin
  1/intake manifold volume : Gain  Gain=1/Coefs.V_intake_man_m3
  Add1 : Sum  Inputs=++-
  Cus_integrator : Subsystem
  Cus_integrator1 : Subsystem
  Cus_integrator2 : Subsystem
  Divide : Product  Inputs=/*
  Divide1 : Product  Inputs=/*
  Divide2 : Product  Inputs=*/
  Fcn : Fcn  Expr=u(3)*(u(2) - u(1)) - u(4)*u(1)
  Fcn1 : Fcn  Expr=u(1)*u(4) +u(2)*u(5) - u(6)*u(3)
  Intake_manifold_vol : Constant  Value=Coefs.V_intake_man_m3
  Mux : Mux
  Mux1 : Mux  Inputs=6
  gamma* R_air : Gain  Gain=const.gamma_air*const.R_specific_air_KJ_per_kg_kelvin
  intake manifold volume 1 : Gain  Gain=Coefs.V_intake_man_m3
  p_in_man_sim : Outport
  T_in_man_sim : Outport  Port=2
  F_in_man_sim : Outport  Port=3
  wires:
  Add1/1 -> 1/intake manifold volume/1
  1/intake manifold volume/1 -> Cus_integrator/1(in)
  [W_throttle] -> Add1/1
  [W_egr_valve] -> Add1/2
  [W_tot_in_engine] -> Add1/3
  Cus_integrator1/1(F1_intake) -> Mux/1, F_in_man_sim/1
  [W_egr_valve] -> Mux/3
  [W_throttle] -> Mux/4
  Mux/1 -> Fcn/1
  intake manifold volume 1/1 -> Divide/1
  Divide/1 -> Cus_integrator1/1(in)
  [W_throttle] -> Mux1/1
  [W_egr_valve] -> Mux1/2
  [W_tot_in_engine] -> Mux1/3
  Fcn/1 -> Divide/2
  Mux1/1 -> Fcn1/1
  Fcn1/1 -> gamma* R_air/1
  gamma* R_air/1 -> Divide2/1
  Divide2/1 -> Cus_integrator2/1(in)
  Divide1/1 -> T_in_man_sim/1, Mux1/6
  Intake_manifold_vol/1 -> Divide2/2
  " R_air1"/1 -> Divide1/1
  Cus_integrator/1(rho_intake) -> intake manifold volume 1/1, " R_air1"/1  "rho_intake"
  Cus_integrator2/1(p_intake) -> Divide1/2, p_in_man_sim/1
  F2_exhaust_sim/1 -> Mux/2
  T_out_IC/1 -> Mux1/4
  T_out_egr_cooler/1 -> Mux1/5
  W_throttle/1 -> [W_throttle]
  W_egr_valve/1 -> [W_egr_valve]
  W_cyl_in/1 -> [W_tot_in_engine]

== system KD_cl_harness_cl_ouports_added/Intercooler/Intercooler ==
  T_out_comp : Inport
  p_out_comp : Inport  Port=2
  T_ambient : Inport  Port=3
  Constant : Constant  Value=Coefs.ICTemp
  MATLAB Function : MATLAB Function  TreatAsAtomicUnit=on
  T_out_IC : Outport
  p_out_IC : Outport  Port=2
  wires:
  Constant/1 -> MATLAB Function/3(ICTempCoefs)
  T_out_comp/1 -> MATLAB Function/1(T_in_IC)
  MATLAB Function/1(T_out_IC) -> T_out_IC/1
  p_out_comp/1 -> p_out_IC/1
  T_ambient/1 -> MATLAB Function/2(T_ambient)

== system KD_cl_harness_cl_ouports_added/NEDC_cycle/Subsystem1 ==
  In1 : Inport
  Rate Limiter : RateLimiter  RisingSlewLimit=1000  FallingSlewLimit=-1000  SampleTimeMode=inherited  InitialCondition=2500
  Unit Delay : UnitDelay  InitialCondition=2500  SampleTime=-1
  Out1 : Outport
  wires:
  Rate Limiter/1 -> Out1/1
  Unit Delay/1 -> Rate Limiter/1
  In1/1 -> Unit Delay/1

== system KD_cl_harness_cl_ouports_added/Turbine/TurbineMap ==
  note: from TC_0605
  omega_turbo_radS : Inport
  p_exhaust_man : Inport  Port=2
  T_ambient : Inport  Port=3
  T_exhaust_man : Inport  Port=4
  u_VGT : Inport  Port=5
  Constant11 : Constant  Value=const.gamma_air
  Constant12 : Constant  Value=const.Engine_Displacement_Volume_m3
  Constant13 : Constant  Value=const.Cp_Air_300K_J_per_kg_per_K
  Constant7 : Constant  Value=const.turbine_diameter
  Constant8 : Constant  Value=Coefs.TurbFlow
  Constant9 : Constant  Value=Coefs.TurbTemp
  Divide : Product  Inputs=*/
  Fcn3 : Fcn  Expr=Coefs.postTurbine(1)*u(1)^2 + Coefs.postTurbine(2)*u(1) + Coefs.postTurbine(3)
  Memory : Memory  X0=IV.W_turbine  InheritSampleTime=on
  Mux3 : Mux
  Terminator_{1..4} (4 alike) : Terminator
  TurbineMAP1 : MATLAB Function  Priority=2  TreatAsAtomicUnit=on
  conversion to RPM : Gain  Gain=30/pi
  W_out_turb_sim : Outport
  T_out_turb_sim : Outport  Port=2
  Tq_turbine : Outport  Port=3
  wires:
  omega_turbo_radS/1 -> conversion to RPM/1
  conversion to RPM/1 -> TurbineMAP1/2(omega_turbo)
  Constant12/1 -> Mux3/4
  Constant11/1 -> Mux3/3
  Constant7/1 -> Mux3/1
  Mux3/1 -> TurbineMAP1/7(Turb_Constants)
  Constant8/1 -> TurbineMAP1/8(TurbFlowCoefs)
  Constant9/1 -> TurbineMAP1/9(TurbTempCoefs)
  TurbineMAP1/1(W_turbine_sim) -> Memory/1, W_out_turb_sim/1
  TurbineMAP1/2(T_out_turbine) -> T_out_turb_sim/1
  TurbineMAP1/7(Tq_turbine) -> Tq_turbine/1
  Divide/1 -> TurbineMAP1/1(turb_pres_ratio)
  Fcn3/1 -> Divide/1
  p_exhaust_man/1 -> TurbineMAP1/3(p_in_turb), Divide/2
  Constant13/1 -> Mux3/2
  Memory/1 -> Fcn3/1
  T_ambient/1 -> TurbineMAP1/4(T_ambient)
  u_VGT/1 -> TurbineMAP1/6(VNlift)
  T_exhaust_man/1 -> TurbineMAP1/5(T_exh_man)
  TurbineMAP1/3(eta_turb) -> Terminator_3/1
  TurbineMAP1/4(A_turbine) -> Terminator_1/1
  TurbineMAP1/5(phi) -> Terminator_2/1
  TurbineMAP1/6(delta_T_Turbo) -> Terminator_4/1

== system KD_cl_harness_cl_ouports_added/Turbo Rotational Dynamics/Turbo rot ==
  note: stop simulation if turbo speed reaches below 1000 rad/sec
  Tq_compressor : Inport
  Tq_turbine : Inport  Port=2
  1/J_turbo : Gain  Gain=1/Coefs.J_turbo
  Compare To Constant : simulink/Logic and Bit Operations/Compare To Constant  relop=<=  const=1000  OutDataTypeStr=boolean
  Cus_integrator : Subsystem
  Stop Simulation : Stop
  Subtract : Sum  Inputs=--+
  To Workspace15 : ToWorkspace  VariableName=Tq_friction  SampleTime=-1
  Tq_friction : Fcn  Expr=Coefs.Tq_fNT(1) * u(1)^2 + Coefs.Tq_fNT(2) * u(1) + Coefs.Tq_fNT(3)
  Omega_turbo_radS : Outport
  wires:
  Subtract/1 -> 1/J_turbo/1
  1/J_turbo/1 -> Cus_integrator/1(delta_torque)
  Cus_integrator/1(NT_radS) -> Tq_friction/1, Compare To Constant/1, Omega_turbo_radS/1  "omega_turbo_radS"
  Tq_compressor/1 -> Subtract/2
  Tq_turbine/1 -> Subtract/3
  Tq_friction/1 -> To Workspace15/1, Subtract/1
  Compare To Constant/1 -> Stop Simulation/1

== system KD_cl_harness_cl_ouports_added/ctrl_rb_explicit_20140220_v6_simp/EGR_max_flow ==
  Ne_rpm : Inport
  fuel : Inport  Port=2
  egr_cons_abs : Inport  Port=3
  Data Store Write13 : DataStoreWrite  DataStoreName=mon_flowmax
  MinMax : MinMax  Inputs=2
      settings: AttributesFormatString=%<Function>
  Saturation : Saturate  UpperLimit=c_fflow_max  LowerLimit=c_fflow_min
      settings: AttributesFormatString=%<LowerLimit>\n%<UpperLimit>
  egr_ecu : Lookup2D  RowIndex=valveinv.fuel_z  ColumnIndex=valveinv.ene_column  Table=valveinv.flowmax  LookUpMeth=Interpolation-Use End Values
      settings: AttributesFormatString=%<LookUpMeth>\n%<RowIndex>\n%<ColumnIndex>\n%<Table>
  mon_flowmax : Gain
  n4 : Gain  Gain=c_1000inv
      settings: AttributesFormatString=%<Gain>
  n6 : Gain  Gain=1000
      settings: AttributesFormatString=%<Gain>
  tokgps1 : Gain  Gain=c_1000inv
  egr_flow_max : Outport  OutDataTypeStr=single
  sat_out-7 : Outport  Port=2
  wires:
  Ne_rpm/1 -> egr_ecu/2
  Saturation/1 -> MinMax/1
  fuel/1 -> egr_ecu/1
  egr_ecu/1 -> tokgps1/1
  tokgps1/1 -> Saturation/1, sat_out-7/1
  n6/1 -> mon_flowmax/1
  n4/1 -> MinMax/2
  MinMax/1 -> n6/1, egr_flow_max/1
  mon_flowmax/1 -> Data Store Write13/1
  egr_cons_abs/1 -> n4/1

== system KD_cl_harness_cl_ouports_added/ctrl_rb_explicit_20140220_v6_simp/HQPKWIK_V6 ==
  u : Inport
  QPKWIK_Main : Subsystem
  Reshape_output : Reshape
  Saturation1 : Saturate  UpperLimit=HQP_saturation  LowerLimit=mHQP_saturation
      settings: AttributesFormatString=%<LowerLimit>\n%<UpperLimit>
  Saturation2 : Saturate  UpperLimit=HQP_saturation  LowerLimit=mHQP_saturation
      settings: AttributesFormatString=%<LowerLimit>\n%<UpperLimit>
  b_extraction : Subsystem
  x0_calculation : Subsystem
  delU : Outport
  SL_sum : Outport  Port=2  InitialOutput=0
  sat_out-8 : Outport  Port=3
  sat_out-9 : Outport  Port=4
  wires:
  b_extraction/1(boutput) -> QPKWIK_Main/1(b)
  x0_calculation/2(c) -> QPKWIK_Main/3(c)
  x0_calculation/1(xout) -> QPKWIK_Main/2(x0)
  u/1 -> Saturation1/1, sat_out-8/1
  QPKWIK_Main/1(controlinput) -> Reshape_output/1
  Reshape_output/1 -> Saturation2/1, sat_out-9/1
  Saturation1/1 -> b_extraction/1(uinput), x0_calculation/1(uinput)
  Saturation2/1 -> delU/1
  QPKWIK_Main/2(SL_sum) -> SL_sum/1

== system KD_cl_harness_cl_ouports_added/ctrl_rb_explicit_20140220_v6_simp/apply_gs ==
  ustar : Inport
  gs1 : Inport  Port=2
  gs2 : Inport  Port=3
  gs3 : Inport  Port=4
  gs4 : Inport  Port=5
  tictoc : Inport  Port=6
  Demux1 : Demux  Outputs=3
  Demux4 : Demux  Outputs=2
  Divide{1..4} (4 alike) : Product  Inputs=**
  Mux8 : Mux  Inputs=2
  Mux9 : Mux  Inputs=2
  Relational Operator4 : RelationalOperator  Operator=>  OutDataTypeStr=boolean
      settings: AttributesFormatString=%<Operator>
  Switch4 : Switch  Criteria=u2 ~= 0
      settings: AttributesFormatString=%<Criteria>
  zerop5 : Constant  Value=0.5  OutDataTypeStr=single  SampleTime=sample_time
      settings: AttributesFormatString=%<Value>\n%<SampleTime>
  delu1 : Outport
  delu2 : Outport  Port=2
  slack : Outport  Port=3
  out-7 : Outport  Port=4
  out-18 : Outport  Port=5
  wires:
  Demux4/2 -> delu2/1
  [u2tic] -> Mux8/2
  [u1tic] -> Mux8/1
  Divide3/1 -> [u1toc]
  Divide1/1 -> [u2toc]
  Divide2/1 -> [u2tic]
  Divide4/1 -> [u1tic]
  gs2/1 -> Divide2/2
  gs1/1 -> Divide4/1
  Demux1/3 -> slack/1
  Demux4/1 -> delu1/1
  Switch4/1 -> Demux4/1
  Mux9/1 -> Switch4/3
  Mux8/1 -> Switch4/1
  [u2toc] -> Mux9/2
  [u1toc] -> Mux9/1
  ustar/1 -> Demux1/1
  zerop5/1 -> Relational Operator4/2
  Relational Operator4/1 -> Switch4/2, out-18/1
  tictoc/1 -> Relational Operator4/1, out-7/1
  Demux1/2 -> Divide2/1, Divide3/1
  Demux1/1 -> Divide4/2, Divide1/1
  gs4/1 -> Divide1/2
  gs3/1 -> Divide3/2

== system KD_cl_harness_cl_ouports_added/ctrl_rb_explicit_20140220_v6_simp/calc_u ==
  tu1max : Inport
  tu1min : Inport  Port=2
  delu : Inport  Port=3
  clff : Inport  Port=4
  tictoc : Inport  Port=5
  tu2max : Inport  Port=6
  tu2min : Inport  Port=7
  Data Store Write18 : DataStoreWrite  DataStoreName=mon_vgt
  Data Store Write19 : DataStoreWrite  DataStoreName=mon_uwegr
  Demux1 : Demux  Outputs=2
  Demux2 : Demux  Outputs=2
  Gain : Gain  Gain=c_flowdiv
      settings: AttributesFormatString=%<Gain>
  Mux3 : Mux  Inputs=2
  Relational Operator15 : RelationalOperator  Operator=>  OutDataTypeStr=boolean
      settings: AttributesFormatString=%<Operator>
  Saturation7 : Saturate  UpperLimit=c_vnliftmax  LowerLimit=c_vnliftmin
      settings: AttributesFormatString=%<LowerLimit>\n%<UpperLimit>
  Saturation_Dynamic2 : simulink/Discontinuities/Saturation Dynamic  OutMin=[]  OutMax=[]  OutDataTypeStr=Inherit: Same as second input  OutDataType=fixdt(1, 16)  OutScaling=2^-10  DoSatur=off
  Saturation_Dynamic3 : simulink/Discontinuities/Saturation Dynamic  OutMin=[]  OutMax=[]  OutDataTypeStr=Inherit: Same as second input  OutDataType=fixdt(1, 16)  OutScaling=2^-10  DoSatur=off
  Sum1 : Sum  Inputs=++|  OutDataTypeStr=single
  Sum14 : Sum  Inputs=++|
  Switch15 : Switch  Criteria=u2 ~= 0
      settings: AttributesFormatString=%<Criteria>
  Unit Delay1 : UnitDelay  InitialCondition=uz_init  SampleTime=-1
      settings: AttributesFormatString=%<X0>
  mon_uwegr : Gain
  mon_vgt : Gain
  n7 : Gain  Gain=1000
      settings: AttributesFormatString=%<Gain>
  zero15 : Constant  Value=0  OutDataTypeStr=single  SampleTime=sample_time
      settings: AttributesFormatString=%<Value>\n%<SampleTime>
  uegrflow : Outport
  uz : Outport  Port=2
  u_unlift : Outport  Port=3
  sat_out-10 : Outport  Port=4
  out-8 : Outport  Port=5
  out-19 : Outport  Port=6
  wires:
  Mux3/1 -> Sum1/2
  Saturation_Dynamic3/1 -> Mux3/2
  Saturation_Dynamic2/1 -> Mux3/1
  Demux1/2 -> Saturation_Dynamic3/2
  Demux1/1 -> Saturation_Dynamic2/2
  Sum1/1 -> Switch15/1, Unit Delay1/1
  Switch15/1 -> Sum14/2
  zero15/1 -> Relational Operator15/2
  Relational Operator15/1 -> Switch15/2, out-19/1
  Sum14/1 -> Demux2/1
  mon_vgt/1 -> Data Store Write18/1
  n7/1 -> mon_uwegr/1
  Unit Delay1/1 -> Sum1/1, uz/1, [uz]
  Gain/1 -> n7/1, uegrflow/1
  Demux2/2 -> Gain/1
  Demux2/1 -> mon_vgt/1, Saturation7/1, sat_out-10/1
  mon_uwegr/1 -> Data Store Write19/1
  tu1max/1 -> Saturation_Dynamic2/1
  tu1min/1 -> Saturation_Dynamic2/3
  delu/1 -> Demux1/1
  Saturation7/1 -> u_unlift/1
  clff/1 -> Sum14/1
  tictoc/1 -> Relational Operator15/1, out-8/1
  tu2max/1 -> Saturation_Dynamic3/1
  tu2min/1 -> Saturation_Dynamic3/3
  [uz] -> Switch15/3

== system KD_cl_harness_cl_ouports_added/ctrl_rb_explicit_20140220_v6_simp/calc_y_constraints ==
  wcylgps : Inport
  map_ref : Inport  Port=2
  wt_to_map_con : Inport  Port=3
  map : Inport  Port=4
  Data Store Read1 : DataStoreRead  DataStoreName=man_map_cons
  Data Store Read17 : DataStoreRead  DataStoreName=man_pex_cons
  Data Store Read4 : DataStoreRead  DataStoreName=man_egrr_cons
  Data Store Write35 : DataStoreWrite  DataStoreName=mon_pex_lead
  Ground1 : Ground
  If1 : If  NumInputs=3  IfExpression=(u1 > u2) | (u1 > u3)  ShowElse=off
  If_Action_Subsystem : Subsystem  TreatAsAtomicUnit=on
  MinMax1 : MinMax  Inputs=2
      settings: AttributesFormatString=%<Function>
  Mux4 : Mux
  Product2 : Product  RndMeth=Zero
  Saturation9 : Saturate  UpperLimit=250  LowerLimit=97  OutDataTypeStr=single
      settings: AttributesFormatString=%<LowerLimit>\n%<UpperLimit>
  Sum19 : Sum  Inputs=|-+
  Sum7 : Sum  Inputs=|-+
  Unit Delay9 : UnitDelay  InitialCondition=250  SampleTime=-1
      settings: AttributesFormatString=%<X0>
  divby100 : Gain  Gain=c_100inv
  dummy1 : Constant  OutDataTypeStr=single  SampleTime=sample_time
      settings: AttributesFormatString=%<Value>\n%<SampleTime>
  man_egrr_cons : Gain
  man_map_cons1 : Gain
  man_pex_cons : Gain
  mon_pex_lead1 : Gain
  egr_cons_abs : Outport
  pex_cons : Outport  Port=2
  y_cons : Outport  Port=3
  map_cons_abs : Outport  Port=4
  sat_out-11 : Outport  Port=5
  wires:
  MinMax1/1 -> Sum7/2
  Saturation9/1 -> Unit Delay9/1, MinMax1/2, mon_pex_lead1/1
  If_Action_Subsystem/1(Out1) -> Saturation9/1, sat_out-11/1
  man_map_cons1/1 -> map_cons_abs/1, [map_cons_abs], Sum19/1
  Sum19/1 -> If1/3
  Unit Delay9/1 -> Sum19/2
  map_ref/1 -> If1/1, Sum7/1, [map_ref]
  If1/1 -> If_Action_Subsystem/Action
  Data Store Read1/1 -> man_map_cons1/1
  mon_pex_lead1/1 -> Data Store Write35/1
  Data Store Read17/1 -> man_pex_cons/1
  man_pex_cons/1 -> pex_cons/1, [pex_cons]
  dummy1/1 -> Mux4/4
  Ground1/1 -> Mux4/2
  divby100/1 -> Product2/1
  Data Store Read4/1 -> man_egrr_cons/1
  man_egrr_cons/1 -> divby100/1
  Product2/1 -> egr_cons_abs/1
  wcylgps/1 -> Product2/2
  Mux4/1 -> y_cons/1
  wt_to_map_con/1 -> MinMax1/1
  map/1 -> If1/2
  Sum7/1 -> Mux4/1
  [map_ref] -> If_Action_Subsystem/2(In2)
  [map_cons_abs] -> If_Action_Subsystem/1(In1)
  [pex_cons] -> Mux4/3

== system KD_cl_harness_cl_ouports_added/ctrl_rb_explicit_20140220_v6_simp/deadzone5 ==
  In1 : Inport
  Abs : Abs
  Divide7 : Product  Inputs=**
  Lookup_Table : Lookup  InputValues=[-1 -.5 -.25 1]  Table=[-1 -1 1 1]
  Saturation : Saturate  UpperLimit=inf  LowerLimit=c_p00001
      settings: AttributesFormatString=%<LowerLimit>\n%<UpperLimit>
  Sign : Signum
  Out1 : Outport
  sat_out-12 : Outport  Port=2
  wires:
  Divide7/1 -> Out1/1
  In1/1 -> Abs/1, Sign/1
  Sign/1 -> Lookup_Table/1
  Saturation/1 -> Divide7/2
  Abs/1 -> Saturation/1, sat_out-12/1
  Lookup_Table/1 -> Divide7/1

== system KD_cl_harness_cl_ouports_added/ctrl_rb_explicit_20140220_v6_simp/deadzone6 ==
  In1 : Inport
  Abs : Abs
  Divide7 : Product  Inputs=**
  Lookup_Table : Lookup  InputValues=[-1 -.5 -.25 1]  Table=[-1 -1 1 1]
  Saturation : Saturate  UpperLimit=inf  LowerLimit=c_p00001
      settings: AttributesFormatString=%<LowerLimit>\n%<UpperLimit>
  Sign : Signum
  Out1 : Outport
  sat_out-13 : Outport  Port=2
  wires:
  Lookup_Table/1 -> Divide7/1
  Abs/1 -> Saturation/1, sat_out-13/1
  Saturation/1 -> Divide7/2
  Sign/1 -> Lookup_Table/1
  In1/1 -> Sign/1, Abs/1
  Divide7/1 -> Out1/1

== system KD_cl_harness_cl_ouports_added/ctrl_rb_explicit_20140220_v6_simp/deadzone7 ==
  In1 : Inport
  Abs : Abs
  Divide7 : Product  Inputs=**
  Lookup_Table : Lookup  InputValues=[-1 -.5 -.25 1]  Table=[-1 -1 1 1]
  Saturation : Saturate  UpperLimit=inf  LowerLimit=c_p00001
      settings: AttributesFormatString=%<LowerLimit>\n%<UpperLimit>
  Sign : Signum
  Out1 : Outport
  sat_out-14 : Outport  Port=2
  wires:
  Divide7/1 -> Out1/1
  In1/1 -> Abs/1, Sign/1
  Sign/1 -> Lookup_Table/1
  Saturation/1 -> Divide7/2
  Abs/1 -> Saturation/1, sat_out-14/1
  Lookup_Table/1 -> Divide7/1

== system KD_cl_harness_cl_ouports_added/ctrl_rb_explicit_20140220_v6_simp/deadzone8 ==
  In1 : Inport
  Abs : Abs
  Divide7 : Product  Inputs=**
  Lookup_Table : Lookup  InputValues=[-1 -.5 -.25 1]  Table=[-1 -1 1 1]
  Saturation : Saturate  UpperLimit=inf  LowerLimit=c_p00001
      settings: AttributesFormatString=%<LowerLimit>\n%<UpperLimit>
  Sign : Signum
  Out1 : Outport
  sat_out-15 : Outport  Port=2
  wires:
  Lookup_Table/1 -> Divide7/1
  Abs/1 -> Saturation/1, sat_out-15/1
  Saturation/1 -> Divide7/2
  Sign/1 -> Lookup_Table/1
  In1/1 -> Sign/1, Abs/1
  Divide7/1 -> Out1/1

== system KD_cl_harness_cl_ouports_added/ctrl_rb_explicit_20140220_v6_simp/deconstruct_vlve_thr ==
  uvalve : Inport
  Data Store Write20 : DataStoreWrite  DataStoreName=mon_valve
  Saturation8 : Saturate  UpperLimit=70  LowerLimit=0  OutDataTypeStr=single
      settings: AttributesFormatString=%<LowerLimit>\n%<UpperLimit>
  Sum11 : Sum  Inputs=|+-
  Unit Delay4 : UnitDelay  SampleTime=-1
      settings: AttributesFormatString=%<X0>
  mon_valve : Gain
  u_throttle : Outport
  u_valve : Outport  Port=2
  valvez : Outport  Port=3
  sat_out-16 : Outport  Port=4
  wires:
  uvalve/1 -> Sum11/1, Saturation8/1, sat_out-16/1
  mon_valve/1 -> Data Store Write20/1
  Saturation8/1 -> Sum11/2, mon_valve/1, Unit Delay4/1, u_valve/1
  Sum11/1 -> u_throttle/1
  Unit Delay4/1 -> valvez/1
